simulink model "MVC_SS"  (R2015b)
settings: Solver=VariableStepAuto  StartTime=0.0  StopTime=10.0  RelTol=1e-3
values from neighbouring files (symbols this model uses):
  A = [-0.313 56.7 0;-0.0139 -0.426 0;0 56.7 0]    [MvcLAB.m]
  Ahat = A    [MvcLAB.m]
  B = [0.232;0.0203;0]    [MvcLAB.m]
  Bhat = [B L]    [MvcLAB.m]
  C = eye(3)    [MvcLAB.m]
  Chat = eye(3)    [MvcLAB.m]
  D = [0;0;0]    [MvcLAB.m]
  Dhat = [0 0;0 0;0 0]    [MvcLAB.m]
  K = place(A,B,J)    [MvcLAB.m]
settings Model: Creator=Satwik  LastModifiedBy=Satwik

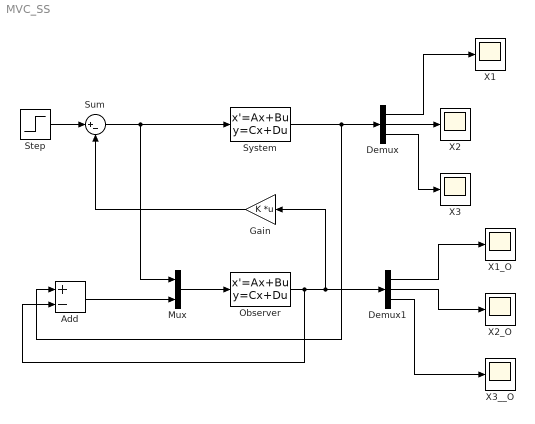
== system MVC_SS ==
  Add : Sum  Inputs=+-
  Demux : Demux  Outputs=3
  Demux1 : Demux  Outputs=3
  Gain : Gain  Gain=K  Multiplication=Matrix(K*u)
  Mux : Mux  Inputs=2
  Observer : StateSpace  A=Ahat  B=Bhat  C=Chat  D=Dhat  X0=0  ContinuousStateAttributes={'X1','X2','X3'}
  Step : Step  Time=0  After=0.2  SampleTime=0
  Sum : Sum  Inputs=|+-
  System : StateSpace  A=A  B=B  C=C  D=D  X0=0  ContinuousStateAttributes={'X1','X2','X3'}
  X1 : Scope
  X1_O : Scope
  X2 : Scope
  X2_O : Scope
  X3 : Scope
  X3__O : Scope
  wires:
  System/1 -> Add/1, Demux/1
  Demux/1 -> X1/1
  Demux/2 -> X2/1
  Demux/3 -> X3/1
  Step/1 -> Sum/1
  Sum/1 -> Mux/1, System/1
  Gain/1 -> Sum/2
  Mux/1 -> Observer/1
  Observer/1 -> Add/2, Gain/1, Demux1/1
  Demux1/1 -> X1_O/1
  Demux1/2 -> X2_O/1
  Demux1/3 -> X3__O/1
  Add/1 -> Mux/2
